simulink library "EV_ASWLibs"  (Simulink 7.3)
settings: Solver=FixedStepDiscrete  StartTime=0.0  StopTime=10.0  FixedStep=0.001  RelTol=1e-3
libraries: simulink x2
settings Model: Creator=ECO-app  LastModifiedBy=hanxl  ModifiedComment=hanxl -- Thu Sep 08 18:11:37 2016 -- Version 1.219

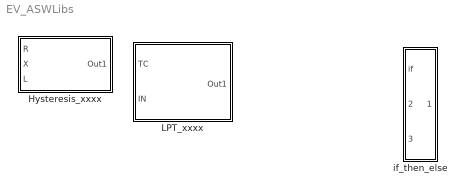
== system EV_ASWLibs ==
  Hysteresis_xxxx : Subsystem  TreatAsAtomicUnit=on
      mask Description:
      | Verson: V0.1
      | AuthorHXL
      | Date:2015-6-29
      | Description
      mask Display:
      | plot([.15 .75 .75 .75 .9],[.15 .15 .15 .85 .85]);
      | plot([.3 .3 .75],[.15 .85 .85]);
      | plot([.25 .3 .35],[.6 .4 .6]);
      | plot([.7 .75 .8],[.4 .6 .4]);
  LPT_xxxx : Subsystem  TreatAsAtomicUnit=on
      settings: RTWFcnNameOpts=Use subsystem name
      mask Description:
      | Verson: V0.1
      | AuthorHXL
      | Date:2015-6-29
      | Description
      mask Display:
      | patch([0 0 1 1], [0 1 1 0], [136/255 136/255 136/255])
      | plot([0 0.30 0.45 0.55 0.63 0.68 0.71 0.74 0.76 0.78  0.795  0.805  0.815 0.82 0.828 0.831 0.832 0.832 0.832 0.832 0.832]);
      | %plot([0:0.1:1],[0 0 0 0.4 0.6 0.7 0.75 0.8 0.825 0.83 0.832]);
      | fprintf('PT1')
      | port_label('input',1,'TC');
      | port_label('input',2,'IN');
  if_then_else : Subsystem
      settings: RTWFcnNameOpts=Use subsystem name  RTWFileNameOpts=Use function name
      mask Description: if then else
      mask Display:
      | %plot([0.2 0.8],[0.9 0.9])
      | %plot([0.3 0.7 1],[0.1 0.5 0.5])
      | %plot([0.8 0.8],[0.55 0.9])
      | %plot([0.75 0.8 0.85],[0.6 0.55 0.6])
      | patch([0 0 1 1], [0 1 1 0], [136/255 136/255 136/255])
      | port_label('input',1,'if')
      | port_label('input',2,'then')
      | port_label('input',3,'else')

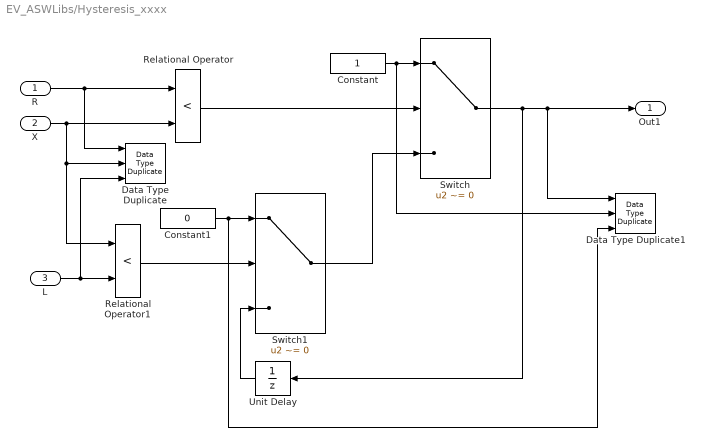
== system EV_ASWLibs/Hysteresis_xxxx ==
  R : Inport
  X : Inport  Port=2
  L : Inport  Port=3
  Constant : Constant  OutDataTypeStr=boolean  OutDataTypeMode=boolean
  Constant1 : Constant  Value=0  OutDataTypeStr=boolean  OutDataTypeMode=boolean
  Data Type Duplicate : simulink/Signal Attributes/Data Type Duplicate  NumInputPorts=3
  Data Type Duplicate1 : simulink/Signal Attributes/Data Type Duplicate  NumInputPorts=3
  Relational Operator : RelationalOperator  Operator=<  OutDataTypeStr=boolean  LogicOutDataTypeMode=boolean
  Relational Operator1 : RelationalOperator  Operator=<  OutDataTypeStr=boolean  LogicOutDataTypeMode=boolean
  Switch : Switch  Criteria=u2 ~= 0
  Switch1 : Switch  Criteria=u2 ~= 0
  Unit Delay : UnitDelay  SampleTime=-1
  Out1 : Outport
  wires:
  Unit Delay/1 -> Switch1/3
  Switch/1 -> Unit Delay/1, Out1/1, Data Type Duplicate1/1
  Constant1/1 -> Data Type Duplicate1/3, Switch1/1
  Relational Operator1/1 -> Switch1/2
  L/1 -> Relational Operator1/2, Data Type Duplicate/3
  Switch1/1 -> Switch/3
  Constant/1 -> Switch/1, Data Type Duplicate1/2
  Relational Operator/1 -> Switch/2
  R/1 -> Relational Operator/1, Data Type Duplicate/1
  X/1 -> Relational Operator/2, Relational Operator1/1, Data Type Duplicate/2

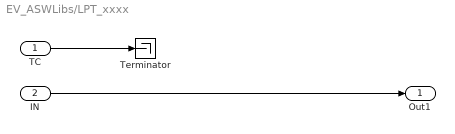
== system EV_ASWLibs/LPT_xxxx ==
  TC : Inport
  IN : Inport  Port=2
  Terminator : Terminator
  Out1 : Outport
  wires:
  TC/1 -> Terminator/1
  IN/1 -> Out1/1

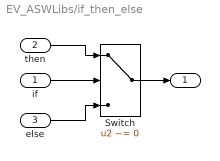
== system EV_ASWLibs/if_then_else ==
  "if    " : Inport
  then : Inport  Port=2
  else : Inport  Port=3
  Switch : Switch  Criteria=u2 ~= 0  Threshold=1  OutDataTypeStr=Inherit: Inherit via back propagation
  " " : Outport
  wires:
  else/1 -> Switch/3
  Switch/1 -> " "/1
  then/1 -> Switch/1
  "if    "/1 -> Switch/2
